simulink model "nonlinear"  (Simulink 7.3)
settings: Solver=ode45  StartTime=0.0  StopTime=130  RelTol=1e-3
values from neighbouring files (symbols this model uses):
  bj = 10    [linear1_param.m]    (also in nonlinear1_param.m = sqrt(10))
  bp = 100    [linear1_param.m]    (also in nonlinear1_param.m = 10)
  g = 9.81    [linear1_param.m]    (also in nonlinear1_param.m)
  k = 400    [linear1_param.m]    (also in nonlinear1_param.m)
  mj = 100    [linear1_param.m]    (also in nonlinear1_param.m)
  mp = 60    [linear1_param.m]    (also in nonlinear1_param.m)
settings Model: Creator=m134506  LastModifiedBy=m134506
settings DebuggingCC: SaveWithParameterizedLinksMsg=none  MultiTaskCondExecSysMsg=none  StrictBusMsg=None
settings RTWCC: IncludeERTFirstTime=on

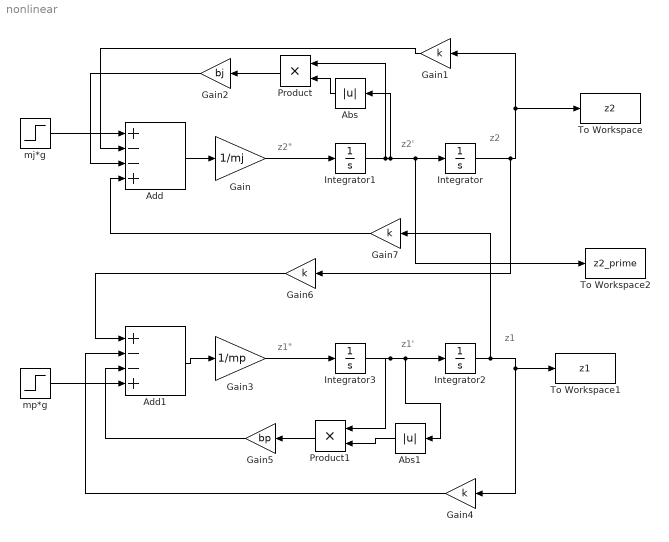
== system nonlinear ==
  note: z2"
  note: z2'
  note: z2
  note: z1"
  note: z1'
  note: z1
  Abs : Abs
  Abs1 : Abs
  Add : Sum  Inputs=+--+  OutDataType=sfix(16)  OutScaling=2^0  OutDataTypeStr=Inherit: Same as first input
  Add1 : Sum  Inputs=+--+  OutDataType=sfix(16)  OutScaling=2^0  OutDataTypeStr=Inherit: Same as first input
  Gain : Gain  Gain=1/mj  ParameterDataType=sfix(16)  ParameterScaling=2^0  OutDataType=sfix(16)  OutScaling=2^0  OutDataTypeStr=Inherit: Same as input  ParamDataTypeStr=Inherit: Same as input
  Gain{1,4,6..7} (4 alike) : Gain  Gain=k  ParameterDataType=sfix(16)  ParameterScaling=2^0  OutDataType=sfix(16)  OutScaling=2^0  OutDataTypeStr=Inherit: Same as input  ParamDataTypeStr=Inherit: Same as input
  Gain2 : Gain  Gain=bj  ParameterDataType=sfix(16)  ParameterScaling=2^0  OutDataType=sfix(16)  OutScaling=2^0  OutDataTypeStr=Inherit: Same as input  ParamDataTypeStr=Inherit: Same as input
  Gain3 : Gain  Gain=1/mp  ParameterDataType=sfix(16)  ParameterScaling=2^0  OutDataType=sfix(16)  OutScaling=2^0  OutDataTypeStr=Inherit: Same as input  ParamDataTypeStr=Inherit: Same as input
  Gain5 : Gain  Gain=bp  ParameterDataType=sfix(16)  ParameterScaling=2^0  OutDataType=sfix(16)  OutScaling=2^0  OutDataTypeStr=Inherit: Same as input  ParamDataTypeStr=Inherit: Same as input
  Integrator : Integrator  InitialCondition=-1250
  Integrator1 : Integrator
  Integrator2 : Integrator  InitialCondition=-1250
  Integrator3 : Integrator
  Product : Product  OutDataType=sfix(16)  OutScaling=2^0  RndMeth=Zero
  Product1 : Product  OutDataType=sfix(16)  OutScaling=2^0  RndMeth=Zero
  To Workspace : ToWorkspace  VariableName=z2  SampleTime=-1  SaveFormat=Array
  To Workspace1 : ToWorkspace  VariableName=z1  SampleTime=-1  SaveFormat=Array
  To Workspace2 : ToWorkspace  VariableName=z2_prime  SampleTime=-1  SaveFormat=Array
  mj*g : Step  After=g*mj  SampleTime=0
  mp*g : Step  After=g*mp  SampleTime=0
  wires:
  Integrator1/1 -> Product/1, Integrator/1, To Workspace2/1, Abs/1
  Gain/1 -> Integrator1/1
  Add/1 -> Gain/1
  mj*g/1 -> Add/1
  Integrator/1 -> Gain6/1, Gain1/1, To Workspace/1
  Gain1/1 -> Add/2
  Gain2/1 -> Add/3
  Integrator3/1 -> Product1/1, Integrator2/1, Abs1/1
  Gain3/1 -> Integrator3/1
  Add1/1 -> Gain3/1
  Gain6/1 -> Add1/1
  Integrator2/1 -> Gain7/1, Gain4/1, To Workspace1/1
  Gain4/1 -> Add1/2
  Gain5/1 -> Add1/3
  Gain7/1 -> Add/4
  Product/1 -> Gain2/1
  Product1/1 -> Gain5/1
  Abs/1 -> Product/2
  Abs1/1 -> Product1/2
  mp*g/1 -> Add1/4
